simulink model "SiMoDronesBebopRos_student"  (R2021a)
settings: Solver=FixedStepAuto  StartTime=0  StopTime=35  FixedStep=0.005  MaxStep=1e-3  MinStep=5e-5  RelTol=1e-5  AbsTol=1e-5
StopFcn:
  | %data_bebop;
  | save_and_plot_data
values from neighbouring files (symbols this model uses):
  aero =     [test1_p1.mat]    (also in test2_P2.mat; test3_pd.mat; test4_lat.mat; xtest4_lat.mat)
  controlGains =     [test1_p1.mat]    (also in test2_P2.mat; test3_pd.mat; test4_lat.mat; xtest4_lat.mat)
  drone =     [test1_p1.mat]    (also in test2_P2.mat; test3_pd.mat; test4_lat.mat; xtest4_lat.mat)
  init_state =     [test1_p1.mat]    (also in test2_P2.mat; test3_pd.mat; test4_lat.mat; xtest4_lat.mat)
  K = place(A,B,P0)    [Control.m]    (also in test1_p1.mat = [0.637104994903 0.356778797146]; test2_P2.mat = [0.637104994903 0.356778797146]; test3_pd.mat = [0.637104994903 0.356778797146]; test4_lat.mat = [0.637104994903 0.356778797146])
  Kd = 3.806    [Control.m]    (also in test1_p1.mat = 5.726; test2_P2.mat = 5.726; test3_pd.mat = 5.726; test4_lat.mat = 5.726)
  Kdd = 2*sg*om*tau-1    (= 0.98)    [Control.m]    (also in test1_p1.mat = 1.509; test2_P2.mat = 1.509; test3_pd.mat; test4_lat.mat = 1.509)
  Ki = 37.39    [Control.m]    (also in test1_p1.mat = 83.71; test2_P2.mat = 83.71; test3_pd.mat = 83.71; test4_lat.mat = 83.71)
  Kp = 25.23    [Control.m]    (also in test1_p1.mat = 43.79; test2_P2.mat = 43.79; test3_pd.mat = 43.79; test4_lat.mat = 43.79)
  Kp1 = 4    [Control.m]    (also in test1_p1.mat; test2_P2.mat; test3_pd.mat; test4_lat.mat)
  Kp2 = 5.2071    [Control.m]    (also in test1_p1.mat; test2_P2.mat; test3_pd.mat; test4_lat.mat)
  Kpd = tau*om^2    (= 6.0612244898)    [Control.m]    (also in test1_p1.mat = 12.82; test2_P2.mat = 12.82; test3_pd.mat; test4_lat.mat = 12.82)
  measure =     [test1_p1.mat]    (also in test2_P2.mat; test3_pd.mat; test4_lat.mat; xtest4_lat.mat)
  motor =     [test1_p1.mat]    (also in test2_P2.mat; test3_pd.mat; test4_lat.mat; xtest4_lat.mat)
  N = K1    [Control.m]    (also in test1_p1.mat = 0.637104994903; test2_P2.mat = 0.637104994903; test3_pd.mat = 0.637104994903; test4_lat.mat = 0.637104994903)
  tau = 0.33    [Control.m]    (also in test1_p1.mat; test2_P2.mat; test3_pd.mat; test4_lat.mat)
  Te = Ts_optitrack    (= 0.02)    [Startup_bebop_ros.m]    (also in test1_p1.mat; test2_P2.mat; test3_pd.mat; test4_lat.mat)
  Te_topics_empty = 0.1    [Startup_bebop_ros.m]    (also in test1_p1.mat; test2_P2.mat; test3_pd.mat; test4_lat.mat)
  Ts_bebop = 5e-3    (= 0.005)    [Startup_bebop_ros.m]    (also in test1_p1.mat; test2_P2.mat; test3_pd.mat; test4_lat.mat)
  Ts_bebop_feedback = 2e-1    (= 0.2)    [Startup_bebop_ros.m]    (also in test1_p1.mat; test2_P2.mat; test3_pd.mat; test4_lat.mat)
  Ts_optitrack = 2e-2    (= 0.02)    [Startup_bebop_ros.m]    (also in test1_p1.mat; test2_P2.mat; test3_pd.mat; test4_lat.mat)
undefined symbols (not defined in the file or in its folder): Angular, DiscIntNeverNeededParam, gcbh, Linear, sigbuilder_block, sldros_modeswitch
libraries: robotlib x15, simulink x9, pid_lib x8, vrlib x5, lib_isae_drones x4, aerolibanimutils x2, sharedtransform x2, aerolibobsolete x1, drones x1
(part 3 of 3)

== stateflow chart SiMoDronesBebopRos_student/BEBOP/Bebop Control/Inner Loop (Parrot)/Bebop onboard control/Chart ==
  state InitMotors
  state TakingOff
    bebop_state=1;
  state Landed
    bebop_state=0;
  state Hovering
    bebop_state=2;
  state Flying
    bebop_state=3;
  state Landing
    bebop_state=4;
  Landing -> Flying [order 2] : [(bebop_tgt.Vz~=0)]
  Hovering -> Flying [order 2] : [(bebop_tgt.roll~=0)||...
      | (bebop_tgt.pitch~=0)||...
      | (bebop_tgt.yaw_rate~=0)||...
      | (bebop_tgt.Vz~=0)]
  Landed -> InitMotors : [(bebop_ctrl.takeoff==1)]
  TakingOff -> Hovering : [bebop_sensors.altitude>1.5]
  InitMotors -> TakingOff : after(0.5,'sec')
  (default) -> Landed
  Flying -> Landing [order 2] : [(bebop_ctrl.land==1)&&...
      | (bebop_ctrl.takeoff==0)]
  Hovering -> Landing [order 1] : [(bebop_ctrl.land==1)&&...
      | (bebop_ctrl.takeoff==0)]
  Flying -> Hovering [order 1] : [(bebop_tgt.roll==0)&&...
      | (bebop_tgt.pitch==0)&&...
      | (bebop_tgt.yaw_rate==0)&&...
      | (bebop_tgt.Vz==0)]
  Landing -> Landed [order 1] : [bebop_sensors.altitude<0.2]
  data: bebop_sensors input Bus: BUS_bebop_sensors; bebop_tgt input; bebop_ctrl input; bebop_state output

== matlab function SiMoDronesBebopRos_student/OPTITRACK/Measure /optitrack_/MATLAB Function ==
  data: in input; out output
function out = fcn(in)
%#codegen

%y = mod(u+pi, 2*pi) - pi;

if (in < -pi) || (pi < in)
    out = in + pi;
    out = mod(out, 2*pi) - pi;
else
    out = in;
end

== matlab function SiMoDronesBebopRos_student/BEBOP/Bebop Control/Inner Loop (Parrot)/Bebop onboard control/Vz control/Subsystem/MATLAB Function1 ==
  data: Vz_ref_in input; Vz_ref_out output; Motor_on output; bebop_state input; altitude input
function [Vz_ref_out,Motor_on] = fcn(Vz_ref_in, bebop_state, altitude)
kp = 1;%proportional gain altitude control

switch bebop_state
    case 0 %landed
        Vz_ref_out=0;
        Motor_on=0;
    case 1 %taking off
        Vz_ref_out=-1.5;
        Motor_on=1;
    case 2 %hovering
%         Vz_ref_out=0;
        Vz_ref_out = -kp*(1.5 - altitude);
        Motor_on=1;
    case 3 %flying
        Vz_ref_out=Vz_ref_in;
        Motor_on=1;
    case 4 %landing
        Vz_ref_out=1;
        Motor_on=1;
    otherwise
        Vz_ref_out=0;
        Motor_on=0;

end

== matlab function SiMoDronesBebopRos_student/OPTITRACK/ROS link + Measure/UDP link/optitrack_pos_vel_uav/Computes velocities/computes_vel ==
  data: pos_OT input; vel_OT output
function vel_OT = compute_vel(pos_OT)
%#codegen

persistent pos_OT_old t_old vel_OT_old

if isempty(pos_OT_old)
    pos_OT_old = pos_OT.Pose.Position;
    t_old = double(pos_OT.Header.Stamp.Nsec)*1e-9;
    vel_OT = [0;0;0];
    vel_OT_old = vel_OT;
else
    pos = pos_OT.Pose.Position;
    t = double(pos_OT.Header.Stamp.Nsec)*1e-9;
    if (t > t_old)
        dt = t - t_old;
        vel_OT =  [pos.X - pos_OT_old.X;...
            pos.Y - pos_OT_old.Y; ...
            pos.Z - pos_OT_old.Z]/dt;
    else
        vel_OT = vel_OT_old;
    end
    
    pos_OT_old = pos_OT.Pose.Position;
    t_old = t;
end

vel_OT_old = vel_OT;

== matlab function SiMoDronesBebopRos_student/JOYSTICK/ROS link + Measure/UDP link/MATLAB Function ==
  data: selected_topic input; offboard output
function offboard = check_offboard(selected_topic)

manual_topic_name = uint8('/joy/cmd_vel');
offboard_topic_name = uint8('/bebop/cmd_vel');

% "selected_topic" is a array which is by default 128 char long, check only
% the size of the topic name
if selected_topic(1:size(manual_topic_name,2)) == manual_topic_name'
    offboard = 0;
elseif selected_topic(1:size(offboard_topic_name,2)) == offboard_topic_name'
    offboard = 1;
else
    offboard = -1;
end
